simulink model "VSC_Grid"  (R2016b)
settings: Solver=VariableStepAuto  StartTime=0.0  StopTime=2  FixedStep=Ts  MaxStep=Ts  RelTol=1e-3  AbsTol=1e-3  EnableMultiTasking=on
undefined symbols (not defined in the file): alpha_PLL, alpha_PQ, DiscIntNeverNeededParam, fmax, fmin, fn, Ib, Kp_CC, Lf, Lf_pu, Rf, Sb, Ts, Vb, Vdcb, wn
libraries: powerlib x10, powerlib_meascontrol x10
Description:
  | Copyright 2008-2016 The MathWorks, Inc.
settings Model: FPTRunName=Active  ExtModeTrigMode=oneshot  ExtModeArmWhenConnect=off  ExtModeAutoUpdateStatusClock=off  Creator=MathWorks  LastModifiedBy=peiyuan
settings DataIOCC: SaveFormat=Array  SignalLoggingSaveFormat=ModelDataLogs  SaveOutput=off  SaveTime=off  SignalLoggingName=sigsOut
settings OptimizationCC: BlockReduction=off  BooleanDataType=off  ExpressionDepthLimit=2147483647  InitFltsAndDblsToZero=on  EfficientMapNaN2IntZero=off  LifeSpan=inf
settings DebuggingCC: SaveWithParameterizedLinksMsg=none  UnderspecifiedInitializationDetection=Classic  MergeDetectMultiDrivingBlocksExec=none  CheckExecutionContextPreStartOutputMsg=on  CheckExecutionContextRuntimeOutputMsg=on  SignalResolutionControl=TryResolveAllWithWarning  MultiTaskDSMMsg=warning  MultiTaskCondExecSysMsg=none  FcnCallInpInsideContextMsg=warning  AllowSymbolicDim=off  StateNameClashWarn=warning  SFUnexpectedBacktrackingDiag=warning  SFNoUnconditionalDefaultTransitionDiag=warning  SFExecutionAtInitializationDiag=none
settings HardwareCC: ProdBitPerPointer=32  ProdBitPerSizeT=32  ProdBitPerPtrDiffT=32  ProdLargestAtomicFloat=None  ProdIntDivRoundTo=Undefined  ProdEndianess=Unspecified  ProdWordSize=32  ProdHWDeviceType=32-bit Generic  TargetUnknown=on
settings ModelReferenceCC: PropagateSignalLabelsOutOfModel=off
settings GRTTargetCC: TargetFcnLib=ansi_tfl_tmw.mat  TargetLangStandard=C89/C90 (ANSI)  GeneratePreprocessorConditionals=Disable all  CombineOutputUpdateFcns=off  GRTInterface=on
settings ConfigComp: CovMetricSettings=dw  CovHtmlReporting=on  CovSaveCumulativeToWorkspaceVar=on  CovSaveSingleToWorkspaceVar=on  CovExternalEMLEnable=off  CovSFcnEnable=off

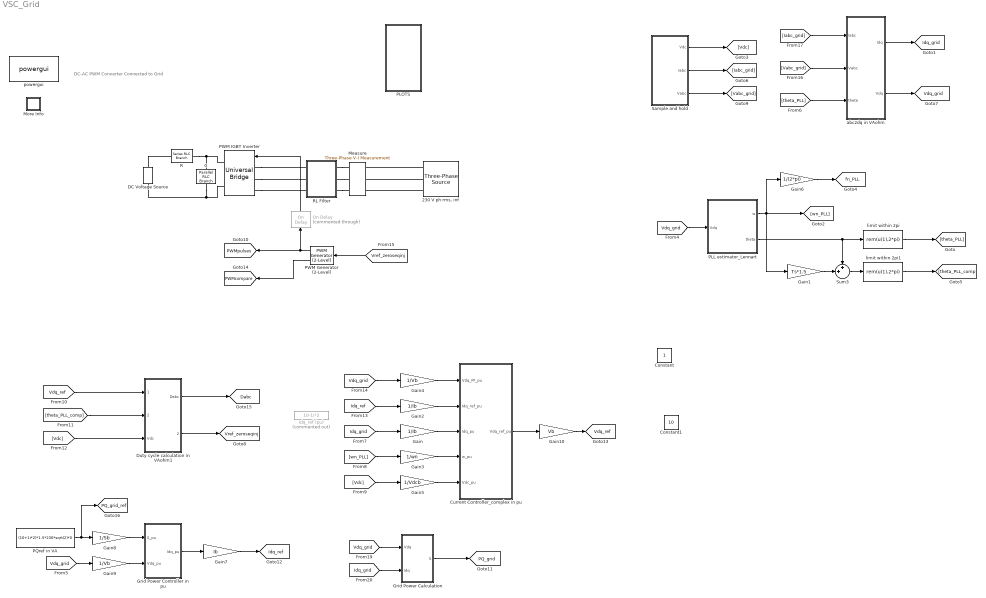
== system VSC_Grid ==
  note: DC-AC PWM Converter Connected to Grid
  "230 V ph rms, inf" : powerlib/Electrical Sources/Three-Phase Source  InternalConnection=Yg  VoltagePhases=off  Voltage=230*sqrt(3)  PhaseAngle=0  Voltage_phases=[25e3 25e3 25e3]/sqrt(3)  PhaseAngles_phases=[0 -120 +120]  Frequency=50  NonIdealSource=off  SpecifyImpedance=on  Resistance=0.8929  Inductance=16.58e-3  ShortCircuitLevel=40e6  BaseVoltage=600  XRratio=7  BusType=swing  Pref=0  Qref=0  Prefabc=[10e3, 10e3, 10e3]  Qrefabc=[0, 0, 0]  Qmin=-inf  Qmax=inf
  C : powerlib/Elements/Parallel RLC Branch  LConnTagsString=a  RConnTagsString=__new0  BranchType=C  Resistance=inf  Inductance=inf  SetiL0=off  InitialCurrent=0  Capacitance=5000e-06  Setx0=off  InitialVoltage=0  Measurements=Branch voltage
  Constant : Constant
  Constant1 : Constant  Value=10
  Current Controller_complex in pu : Subsystem
  DC Voltage Source : powerlib/Electrical Sources/DC Voltage Source  Amplitude=680  Measurements=None
  Duty cycle calculation in VAohm1 : Subsystem
  Gain : Gain  Gain=1/Ib
  Gain1 : Gain  Gain=Ts*1.5
  Gain10 : Gain  Gain=Vb
  Gain2 : Gain  Gain=1/Ib
  Gain3 : Gain  Gain=1/wn
  Gain4 : Gain  Gain=1/Vb
  Gain5 : Gain  Gain=1/Vdcb
  Gain6 : Gain  Gain=1/(2*pi)
  Gain7 : Gain  Gain=Ib
  Gain8 : Gain  Gain=1/Sb
  Gain9 : Gain  Gain=1/Vb
  Grid Power Calculation : Subsystem
  Grid Power Controller in pu : Subsystem
  Idq_ref (pu) : Constant  Commented=on  Value=10-1i*2
  Measure : powerlib/Measurements/Three-Phase V-I Measurement  VoltageMeasurement=phase-to-ground  SetLabelV=on  LabelV=Vabc_grid_analog  Vpu=off  VpuLL=off  CurrentMeasurement=yes  SetLabelI=on  LabelI=Iabc_grid_analog  Ipu=off  Pbase=Sb  Vbase=Vb*sqrt(3/2)  OutputType=Magnitude  PhasorSimulation=off  PSBequivalent=0
  More Info : Subsystem
      settings: OpenFcn=showdemo(bdroot(gcb))
      mask Display: disp('?')
  On Delay : powerlib_meascontrol/Logic/On Delay  Commented=through  DelayType=On delay  delay=0.01  ic=0  Ts=Ts
  PLL estimator_Lennart : Subsystem  mask(PLL estimator (discrete)){alpha_theta=alpha_PLL, fnmax=fmax, fnmin=fmin, f0=fn, Ts=Ts}
      mask prompts: alpha_theta "Bandwidth (natural freq, rad/s)"; fnmax "Max frequency (Hz)"; fnmin "Min frequency (Hz)"; f0 "Initial frequency (Hz)"; Ts "Sampling time (s)"
      mask help: The PLL is implemented according to Harnefors' paper, a second order system with critically damped case (damping ratio =1)
  PLOTS : Subsystem
  PQref in VA : Constant  Value=(10+1i*2)*1.5*230*sqrt(2)*0
  PWM IGBT Inverter : powerlib/Power Electronics/Universal Bridge  Arms=3  SnubberResistance=5000  SnubberCapacitance=inf  Device=IGBT / Diodes  Ron=1e-3  Lon=0  ForwardVoltages="[  0.0  0.0  ]"  ForwardVoltage=.8  GTOparameters=[ 1e-6 ,1e-6 ]  IGBTparameters=[ 1e-6 , 2e-6 ]  Measurements=All voltages and currents  Measurements_2=None  converterType=Rectifier
  PWM Generator (2-Level) : powerlib_meascontrol/Pulse & Signal Generators/PWM Generator (2-Level)  ModulatorType=Three-phase bridge (6 pulses)  ModulatorMode=Unsynchronized  Fc=5000  Pc=0  nF=27  MinMax="[ -1  1 ]"  SamplingTechnique=Symmetrical regular (single edge)  ModulatingSignals=off  m=0.8  Freq=60  Phase=0  Ts=0  ShowCarrierOutport=on
  R : powerlib/Elements/Series RLC Branch  LConnTagsString=__new0  RConnTagsString=__new0  BranchType=R  Resistance=1e-5  Inductance=1e-3  SetiL0=off  InitialCurrent=0  Capacitance=1e-6  Setx0=off  InitialVoltage=0  Measurements=None
  RL Filter : Subsystem
  Sample and hold : Subsystem
  Sum3 : Sum  Inputs=++|  SaturateOnIntegerOverflow=on  InputSameDT=on  OutDataTypeStr=Inherit: Same as first input
  abc2dq in VAohm : Subsystem
  limit within 2pi : Fcn  Expr=rem(u(1),2*pi)
  limit within 2pi1 : Fcn  Expr=rem(u(1),2*pi)
  powergui : powerlib/powergui  Priority=1  SimulationMode=Continuous  SolverType=Tustin/Backward Euler (TBE)  SampleTime=50e-6  frequency=60  SPID=off  DisableSnubberDevices=off  DisableRonSwitches=off  DisableVfSwitches=off  SwTol=0  DisplayEquations=off  Interpol=off  ExternalGateDelay=off  methode=off  Ts=10  FunctionMessages=off  echomessages=off  HookPort=off  EnableUseOfTLC=off  x0status=blocks  frequencyindice=50  Pbase=35e3  ErrMax=1e-4  Iterations=50  UnitsV=V  UnitsW=kW  buscounter=0  RestoreLinks=warning  ResistiveCurrentMeasurement=off  Frange=[0:2:500]  Ylog=off  Xlog=on  ShowGrid=off  save=off  variable=ZData  structure=0  ZoomFFT=off  StartTime=0.0  cycles=1  DisplayStyle=1  fundamental=60  FreqAxis=off  MaxFrequency=1000  frequencyindicesteady=1  RmsSteady=1  display=off
  tag scope: Dabc=global, Idq_grid=global, Idq_ref=global, PQ_grid=global, PQ_grid_ref=global, PWMcompare=global, PWMpulses=global, Vdq_grid=global, Vdq_ref=global, Vref_zeroseqinj=global, fn_PLL=global
  wires:
  On Delay/1 -> PWM IGBT Inverter/1
  PLL estimator_Lennart/2(theta) -> Sum3/1, limit within 2pi/1
  limit within 2pi/1 -> [theta_PLL]
  abc2dq in VAohm/1(Idq) -> [Idq_grid]
  [Vdq_grid] -> Gain4/1
  [Idq_grid] -> Gain/1
  [wn_PLL] -> Gain3/1
  [Vdc] -> Gain5/1
  Current Controller_complex in pu/1(Vdq_ref_pu) -> Gain10/1
  Gain1/1 -> Sum3/2
  Sum3/1 -> limit within 2pi1/1
  limit within 2pi1/1 -> [theta_PLL_comp]
  abc2dq in VAohm/2(Vdq) -> [Vdq_grid]
  [Vref_zeroseqinj] -> PWM Generator (2-Level)/1
  [Vdq_ref] -> Duty cycle calculation in VAohm1/1(Vdq_ref)
  [theta_PLL_comp] -> Duty cycle calculation in VAohm1/2(theta_comp)
  [Vdc] -> Duty cycle calculation in VAohm1/3(Vdc)
  Duty cycle calculation in VAohm1/1(Dabc) -> [Dabc]
  Duty cycle calculation in VAohm1/2(Vref_pu) -> [Vref_zeroseqinj]
  Gain3/1 -> Current Controller_complex in pu/4(w_pu)
  Gain/1 -> Current Controller_complex in pu/3(Idq_pu)
  Gain5/1 -> Current Controller_complex in pu/5(Vdc_pu)
  [theta_PLL] -> abc2dq in VAohm/3(theta)
  Gain4/1 -> Current Controller_complex in pu/1(Vdq_FF_pu)
  [Vdq_grid] -> PLL estimator_Lennart/1(Vdq)
  PLL estimator_Lennart/1(w) -> Gain6/1, Gain1/1, [wn_PLL]
  [Iabc_grid] -> abc2dq in VAohm/1(Iabc)
  [Vabc_grid] -> abc2dq in VAohm/2(Vabc)
  Gain6/1 -> [fn_PLL]
  Sample and hold/2(Iabc) -> [Iabc_grid]
  Sample and hold/3(Vabc) -> [Vabc_grid]
  PQref in VA/1 -> [PQ_grid_ref], Gain8/1
  [Vdq_grid] -> Gain9/1
  Gain8/1 -> Grid Power Controller in pu/1(S_pu)
  Gain9/1 -> Grid Power Controller in pu/2(Vdq_pu)
  Grid Power Controller in pu/1(Idq_pu) -> Gain7/1
  [Vdq_grid] -> Grid Power Calculation/1(Vdq)
  Grid Power Calculation/1(S) -> [PQ_grid]
  [Idq_grid] -> Grid Power Calculation/2(Idq)
  Gain7/1 -> [Idq_ref]
  Gain10/1 -> [Vdq_ref]
  Gain2/1 -> Current Controller_complex in pu/2(Idq_ref_pu)
  [Idq_ref] -> Gain2/1
  PWM Generator (2-Level)/1 -> [PWMpulses], On Delay/1
  PWM Generator (2-Level)/2 -> [PWMcompare]
  Sample and hold/1(Vdc) -> [Vdc]
  connections:
  PWM IGBT Inverter/RConn2 -- DC Voltage Source/LConn1 -- C/RConn1
  R/RConn1 -- C/LConn1 -- PWM IGBT Inverter/RConn1
  RL Filter/RConn1 -- Measure/LConn1
  Measure/LConn2 -- RL Filter/RConn2
  RL Filter/RConn3 -- Measure/LConn3
  PWM IGBT Inverter/LConn2 -- RL Filter/LConn2
  PWM IGBT Inverter/LConn3 -- RL Filter/LConn3
  PWM IGBT Inverter/LConn1 -- RL Filter/LConn1
  "230 V ph rms, inf"/RConn2 -- Measure/RConn2
  "230 V ph rms, inf"/RConn1 -- Measure/RConn1
  R/LConn1 -- DC Voltage Source/RConn1
  "230 V ph rms, inf"/RConn3 -- Measure/RConn3

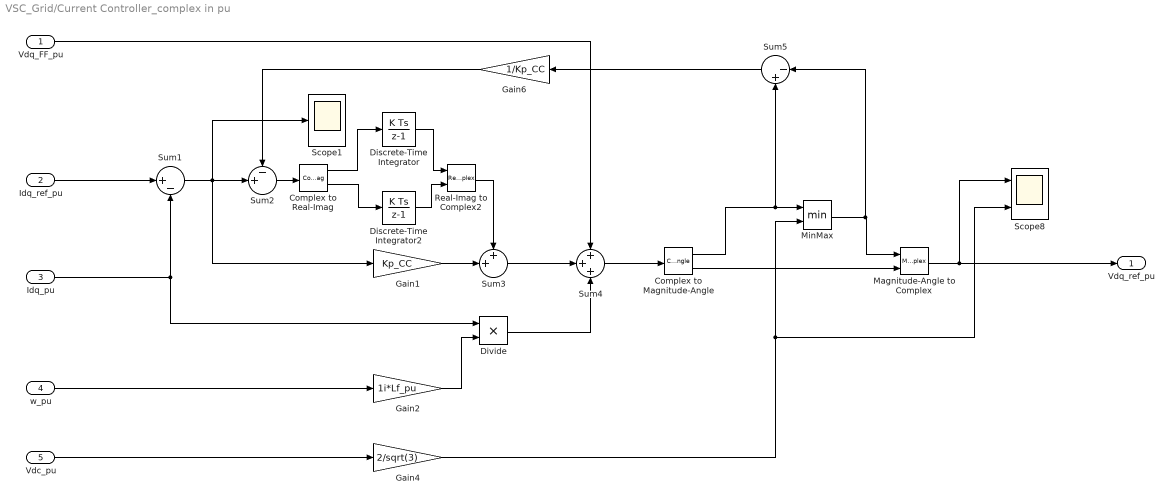
== system VSC_Grid/Current Controller_complex in pu ==
  Vdq_FF_pu : Inport
  Idq_ref_pu : Inport  Port=2
  Idq_pu : Inport  Port=3
  w_pu : Inport  Port=4
  Vdc_pu : Inport  Port=5
  Complex to Magnitude-Angle : ComplexToMagnitudeAngle
  Complex to Real-Imag : ComplexToRealImag
  Discrete-Time Integrator : DiscreteIntegrator  gainval=Ki_CC  InitialConditionSetting=State (most efficient)  SampleTime=Ts  ICPrevOutput=DiscIntNeverNeededParam  ICPrevScaledInput=DiscIntNeverNeededParam
  Discrete-Time Integrator2 : DiscreteIntegrator  gainval=Ki_CC  InitialConditionSetting=State (most efficient)  SampleTime=Ts  ICPrevOutput=DiscIntNeverNeededParam  ICPrevScaledInput=DiscIntNeverNeededParam
  Divide : Product  Inputs=**
  Gain1 : Gain  Gain=Kp_CC
  Gain2 : Gain  Gain=1i*Lf_pu
  Gain4 : Gain  Gain=2/sqrt(3)
  Gain6 : Gain  Gain=1/Kp_CC
  Magnitude-Angle to Complex : MagnitudeAngleToComplex
  MinMax : MinMax  Inputs=2
  Real-Imag to Complex2 : RealImagToComplex
  Scope1 : Scope
  Scope8 : Scope  NumInputPorts=2
  Sum1 : Sum  Inputs=|+-  SaturateOnIntegerOverflow=on  InputSameDT=on  OutDataTypeStr=Inherit: Same as first input
  Sum2 : Sum  Inputs=-+|  SaturateOnIntegerOverflow=on  InputSameDT=on  OutDataTypeStr=Inherit: Same as first input
  Sum3 : Sum  Inputs=++|  SaturateOnIntegerOverflow=on  InputSameDT=on  OutDataTypeStr=Inherit: Same as first input
  Sum4 : Sum  Inputs=+++  SaturateOnIntegerOverflow=on  InputSameDT=on  OutDataTypeStr=Inherit: Same as first input
  Sum5 : Sum  Inputs=|-+  SaturateOnIntegerOverflow=on  InputSameDT=on  OutDataTypeStr=Inherit: Same as first input
  Vdq_ref_pu : Outport
  wires:
  Discrete-Time Integrator2/1 -> Real-Imag to Complex2/2
  Discrete-Time Integrator/1 -> Real-Imag to Complex2/1
  Complex to Real-Imag/2 -> Discrete-Time Integrator2/1
  Real-Imag to Complex2/1 -> Sum3/1
  Complex to Magnitude-Angle/2 -> Magnitude-Angle to Complex/2
  Sum5/1 -> Gain6/1
  Gain4/1 -> Scope8/2, MinMax/2
  Complex to Real-Imag/1 -> Discrete-Time Integrator/1
  Idq_pu/1 -> Divide/1, Sum1/2
  Divide/1 -> Sum4/3
  Idq_ref_pu/1 -> Sum1/1
  Sum4/1 -> Complex to Magnitude-Angle/1
  Sum1/1 -> Scope1/1, Gain1/1, Sum2/2
  Gain2/1 -> Divide/2
  Complex to Magnitude-Angle/1 -> Sum5/2, MinMax/1
  Gain1/1 -> Sum3/2
  Sum3/1 -> Sum4/2
  w_pu/1 -> Gain2/1
  Vdq_FF_pu/1 -> Sum4/1
  Magnitude-Angle to Complex/1 -> Vdq_ref_pu/1, Scope8/1
  Sum2/1 -> Complex to Real-Imag/1
  MinMax/1 -> Sum5/1, Magnitude-Angle to Complex/1
  Gain6/1 -> Sum2/1
  Vdc_pu/1 -> Gain4/1

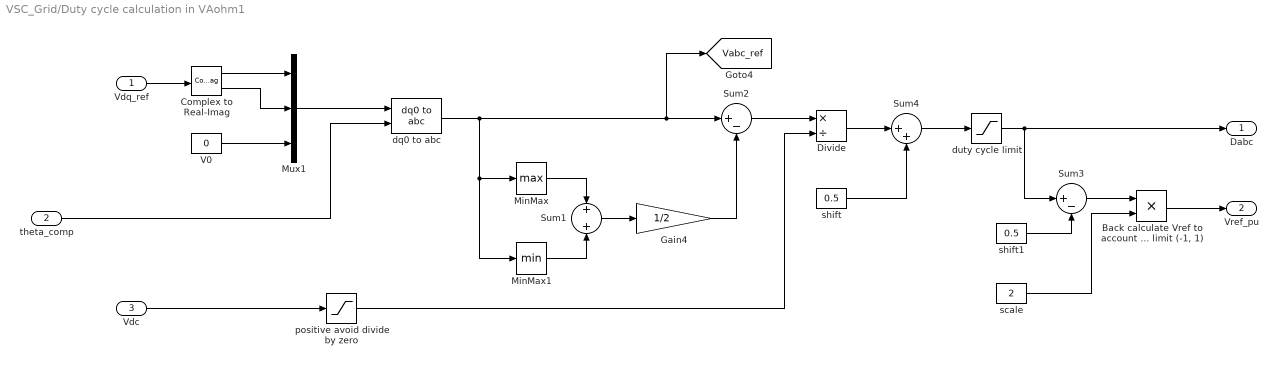
== system VSC_Grid/Duty cycle calculation in VAohm1 ==
  Vdq_ref : Inport
  theta_comp : Inport  Port=2
  Vdc : Inport  Port=3
  "Back calculate Vref to account for duty cycle limit (-1, 1)" : Product  Inputs=**
  Complex to Real-Imag : ComplexToRealImag
  Divide : Product  Inputs=*/
  Gain4 : Gain  Gain=1/2
  MinMax : MinMax  Function=max
  MinMax1 : MinMax
  Mux1 : Mux  Inputs=3
  Sum1 : Sum  SaturateOnIntegerOverflow=on  InputSameDT=on  OutDataTypeStr=Inherit: Same as first input
  Sum2 : Sum  Inputs=|+-  SaturateOnIntegerOverflow=on  InputSameDT=on  OutDataTypeStr=Inherit: Same as first input
  Sum3 : Sum  Inputs=|+-  SaturateOnIntegerOverflow=on  InputSameDT=on  OutDataTypeStr=Inherit: Same as first input
  Sum4 : Sum  Inputs=|++  SaturateOnIntegerOverflow=on  InputSameDT=on  OutDataTypeStr=Inherit: Same as first input
  V0 : Constant  Value=0
  dq0 to abc : powerlib_meascontrol/Transformations/dq0 to abc  Alignment=90 degrees behind phase A axis
  duty cycle limit : Saturate  UpperLimit=0.999  LowerLimit=0.001
  positive avoid divide by zero : Saturate  UpperLimit=inf  LowerLimit=1e-6
  scale : Constant  Value=2
  shift : Constant  Value=0.5
  shift1 : Constant  Value=0.5
  Dabc : Outport
  Vref_pu : Outport  Port=2
  tag scope: Vabc_ref=global
  wires:
  Sum2/1 -> Divide/1
  Gain4/1 -> Sum2/2
  dq0 to abc/1 -> MinMax/1, MinMax1/1, [Vabc_ref], Sum2/1
  MinMax1/1 -> Sum1/2
  shift/1 -> Sum4/2
  Vdq_ref/1 -> Complex to Real-Imag/1
  Complex to Real-Imag/2 -> Mux1/2
  Mux1/1 -> dq0 to abc/1
  Sum1/1 -> Gain4/1
  Divide/1 -> Sum4/1
  Vdc/1 -> positive avoid divide by zero/1
  theta_comp/1 -> dq0 to abc/2
  V0/1 -> Mux1/3
  MinMax/1 -> Sum1/1
  Complex to Real-Imag/1 -> Mux1/1
  Sum4/1 -> duty cycle limit/1
  duty cycle limit/1 -> Sum3/1, Dabc/1
  shift1/1 -> Sum3/2
  Sum3/1 -> "Back calculate Vref to account for duty cycle limit (-1, 1)"/1
  "Back calculate Vref to account for duty cycle limit (-1, 1)"/1 -> Vref_pu/1
  positive avoid divide by zero/1 -> Divide/2
  scale/1 -> "Back calculate Vref to account for duty cycle limit (-1, 1)"/2

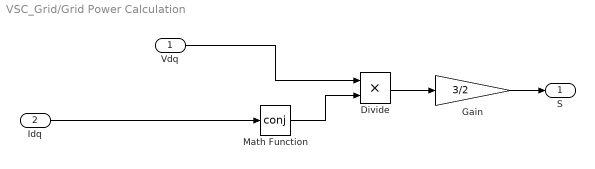
== system VSC_Grid/Grid Power Calculation ==
  Vdq : Inport
  Idq : Inport  Port=2
  Divide : Product  Inputs=**
  Gain : Gain  Gain=3/2
  Math Function : Math  Operator=conj  SaturateOnIntegerOverflow=on
  S : Outport
  wires:
  Idq/1 -> Math Function/1
  Math Function/1 -> Divide/2
  Divide/1 -> Gain/1
  Vdq/1 -> Divide/1
  Gain/1 -> S/1

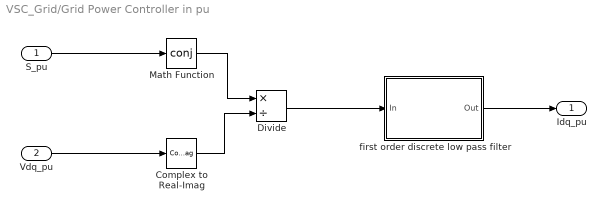
== system VSC_Grid/Grid Power Controller in pu ==
  S_pu : Inport
  Vdq_pu : Inport  Port=2
  Complex to Real-Imag : ComplexToRealImag  Output=Real
  Divide : Product  Inputs=*/
  Math Function : Math  Operator=conj  SaturateOnIntegerOverflow=on
  first order discrete low pass filter : Subsystem  mask(First-order low pass filter (Discrete)){alpha_wfilter=alpha_PQ, Ts=Ts, Init=(10-1i*2)/Ib*0}
      mask prompts: alpha_wfilter "Bandwidth (rad/s)"; Ts "Sampling time (>0, s)"; Init "Initial condition"
      mask help: Forward Euler method
  Idq_pu : Outport
  wires:
  Vdq_pu/1 -> Complex to Real-Imag/1
  Complex to Real-Imag/1 -> Divide/2
  S_pu/1 -> Math Function/1
  Math Function/1 -> Divide/1
  Divide/1 -> first order discrete low pass filter/1(In)
  first order discrete low pass filter/1(Out) -> Idq_pu/1

== system VSC_Grid/More Info ==

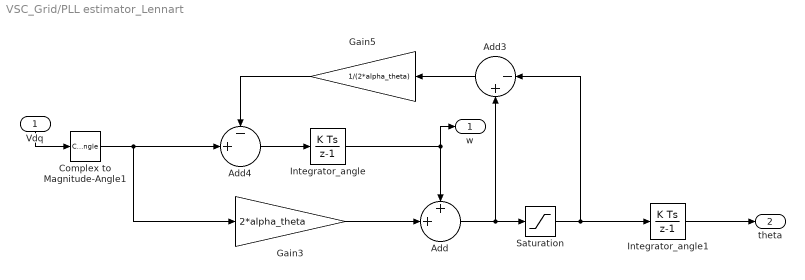
== system VSC_Grid/PLL estimator_Lennart ==
  Vdq : Inport
  Add : Sum  Inputs=++|
  Add3 : Sum  Inputs=|-+
  Add4 : Sum  Inputs=-+|
  Complex to Magnitude-Angle1 : ComplexToMagnitudeAngle  Output=Angle
  Gain3 : Gain  Gain=2*alpha_theta
  Gain5 : Gain  Gain=1/(2*alpha_theta)
  Integrator_angle : DiscreteIntegrator  gainval=alpha_theta^2  InitialCondition=2*pi*f0  InitialConditionSetting=State (most efficient)  SampleTime=Ts  ICPrevOutput=DiscIntNeverNeededParam  ICPrevScaledInput=DiscIntNeverNeededParam
  Integrator_angle1 : DiscreteIntegrator  gainval=1  InitialConditionSetting=State (most efficient)  SampleTime=Ts  ICPrevOutput=DiscIntNeverNeededParam  ICPrevScaledInput=DiscIntNeverNeededParam
  Saturation : Saturate  UpperLimit=2*pi*fnmax  LowerLimit=2*pi*fnmin
  w : Outport
  theta : Outport  Port=2
  wires:
  Integrator_angle1/1 -> theta/1
  Gain5/1 -> Add4/1
  Gain3/1 -> Add/2
  Add/1 -> Add3/2, Saturation/1
  Vdq/1 -> Complex to Magnitude-Angle1/1
  Integrator_angle/1 -> w/1, Add/1
  Add3/1 -> Gain5/1
  Add4/1 -> Integrator_angle/1
  Saturation/1 -> Integrator_angle1/1, Add3/1
  Complex to Magnitude-Angle1/1 -> Gain3/1, Add4/2

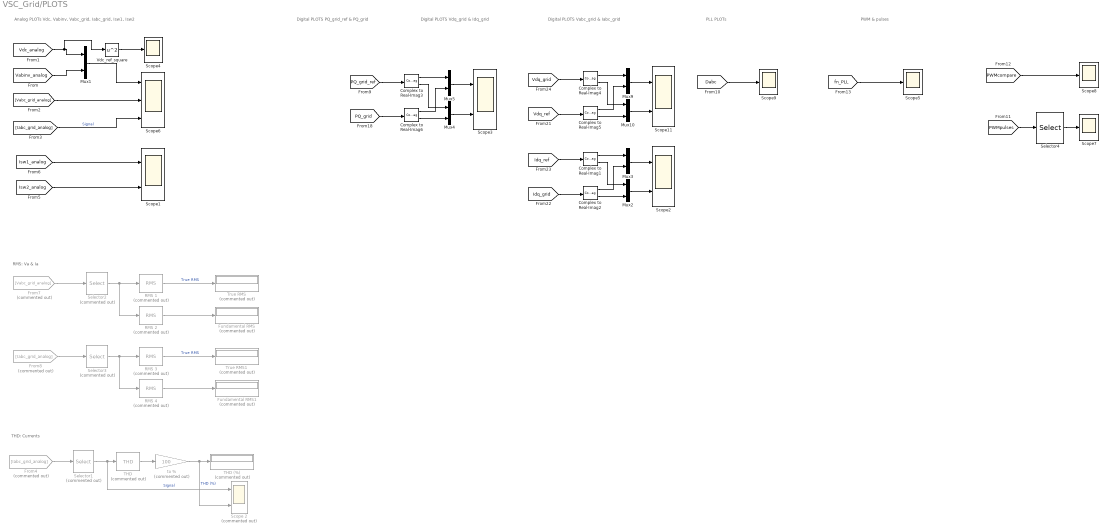
== system VSC_Grid/PLOTS ==
  note: Digital PLOTS
      | Vdq_grid & Idq_grid
  note: Analog PLOTs
      | Vdc, Vabinv, Vabc_grid, Iabc_grid, Isw1, Isw2
  note: THD: Currents
  note: RMS: Va & Ia
  note: PLL PLOTs
  note: Digital PLOTS
      | Vabc_grid & Iabc_grid
  note: PWM & pulses
  note: Digital PLOTS
      | PQ_grid_ref & PQ_grid
  Complex to Real-Imag{1..6} (6 alike) : ComplexToRealImag
  From4 : From  Commented=on  GotoTag=Iabc_grid_analog  TagVisibility=global
  From7 : From  Commented=on  GotoTag=Vabc_grid_analog  TagVisibility=global
  From8 : From  Commented=on  GotoTag=Iabc_grid_analog  TagVisibility=global
  Fundamental RMS : Display  Commented=on
      settings: Format=bank
  Fundamental RMS1 : Display  Commented=on
      settings: Format=bank
  Mux{1..5,9..10} (7 alike) : Mux  Inputs=2
  RMS 1 : powerlib_meascontrol/Measurements/RMS  Commented=on  TrueRMS=on  Freq=fn  RMSInit=Vb  Ts=0
  RMS 2 : powerlib_meascontrol/Measurements/RMS  Commented=on  TrueRMS=off  Freq=fn  RMSInit=Vb  Ts=0
  RMS 3 : powerlib_meascontrol/Measurements/RMS  Commented=on  TrueRMS=on  Freq=fn  RMSInit=Ib  Ts=0
  RMS 4 : powerlib_meascontrol/Measurements/RMS  Commented=on  TrueRMS=off  Freq=fn  RMSInit=Ib  Ts=0
  Scope 2 : Scope  Commented=on  NumInputPorts=2
  Scope{1..3,11} (4 alike) : Scope  NumInputPorts=2
  Scope{4..5,7..9} (5 alike) : Scope
  Scope6 : Scope  NumInputPorts=3
  Selector1 : Selector  Commented=on  InputPortWidth=3  IndexOptions=Index vector (dialog)  Indices=[1]  OutputSizes=1
  Selector2 : Selector  Commented=on  InputPortWidth=3  IndexOptions=Index vector (dialog)  Indices=[1]  OutputSizes=1
  Selector3 : Selector  Commented=on  InputPortWidth=3  IndexOptions=Index vector (dialog)  Indices=[1]  OutputSizes=1
  Selector4 : Selector  InputPortWidth=6  IndexOptions=Index vector (dialog)  Indices=[1]  OutputSizes=1
  THD : powerlib_meascontrol/Measurements/THD  Commented=on  Freq=50  Ts=0
  THD (%) : Display  Commented=on
      settings: Format=bank
  True RMS : Display  Commented=on
      settings: Format=bank
  True RMS1 : Display  Commented=on
      settings: Format=bank
  Vdc_ref_square : Math  Operator=square  SaturateOnIntegerOverflow=on
  to % : Gain  Commented=on  Gain=100  SampleTime=Ts
  wires:
  [Iabc_grid_analog] -> Scope6/3  "Signal"
  to %/1 -> THD (%)/1, Scope 2/2  "THD (%)"
  THD/1 -> to %/1
  [Vdc_analog] -> Vdc_ref_square/1, Mux1/1
  [Vabinv_analog] -> Mux1/2
  Mux1/1 -> Scope6/1
  [Vabc_grid_analog] -> Scope6/2
  [Isw1_analog] -> Scope1/1
  [Isw2_analog] -> Scope1/2
  From4/1 -> Selector1/1
  Selector1/1 -> THD/1, Scope 2/1  "Signal"
  RMS 1/1 -> True RMS/1  "True RMS"
  From7/1 -> Selector2/1
  Selector2/1 -> RMS 2/1, RMS 1/1
  RMS 2/1 -> Fundamental RMS/1
  RMS 3/1 -> True RMS1/1  "True RMS"
  Selector3/1 -> RMS 4/1, RMS 3/1
  RMS 4/1 -> Fundamental RMS1/1
  From8/1 -> Selector3/1
  Vdc_ref_square/1 -> Scope4/1
  [fn_PLL] -> Scope5/1
  [Dabc] -> Scope9/1
  Selector4/1 -> Scope7/1
  [PWMpulses] -> Selector4/1
  [PWMcompare] -> Scope8/1
  Complex to Real-Imag4/1 -> Mux9/1
  Complex to Real-Imag5/1 -> Mux9/2
  Complex to Real-Imag4/2 -> Mux10/1
  Complex to Real-Imag5/2 -> Mux10/2
  Mux9/1 -> Scope11/1
  Mux10/1 -> Scope11/2
  Complex to Real-Imag1/1 -> Mux3/1
  Complex to Real-Imag2/1 -> Mux3/2
  Complex to Real-Imag1/2 -> Mux2/1
  Complex to Real-Imag2/2 -> Mux2/2
  Mux3/1 -> Scope2/1
  Mux2/1 -> Scope2/2
  [Idq_ref] -> Complex to Real-Imag1/1
  [Idq_grid] -> Complex to Real-Imag2/1
  [Vdq_grid] -> Complex to Real-Imag4/1
  [Vdq_ref] -> Complex to Real-Imag5/1
  Complex to Real-Imag3/1 -> Mux5/1
  Complex to Real-Imag6/1 -> Mux5/2
  Complex to Real-Imag3/2 -> Mux4/1
  Complex to Real-Imag6/2 -> Mux4/2
  Mux5/1 -> Scope3/1
  Mux4/1 -> Scope3/2
  [PQ_grid_ref] -> Complex to Real-Imag3/1
  [PQ_grid] -> Complex to Real-Imag6/1

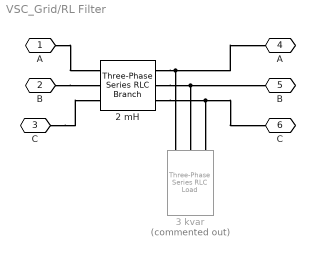
== system VSC_Grid/RL Filter ==
  "2 mH " : powerlib/Elements/Three-Phase Series RLC Branch  LConnTagsString=A|B|C  RConnTagsString=A|B|C  BranchType=RL  Resistance=Rf  Inductance=Lf  Capacitance=inf  Measurements=None
  3 kvar : powerlib/Elements/Three-Phase Series RLC Load  Commented=on  LConnTagsString=A|B|C  Configuration=Y (grounded)  NominalVoltage=380  Vabc=[1e3 1e3 1e3]  Vabcp=[1e3 1e3 1e3]  NominalFrequency=50  UnbalancedPower=off  ActivePower=0  InductivePower=0  CapacitivePower=3e3  Pabc=[10e3 9e3 11e3]  QLabc=[100 90 110]  QCabc=[100 90 110]  Pabcp=[10e3 9e3 11e3]  QLabcp=[100 90 110]  QCabcp=[100 90 110]  Measurements=None  LoadType=constant Z
  A : PMIOPort  Port=1  Side=Left
  B : PMIOPort  Port=2  Side=Left
  C : PMIOPort  Port=3  Side=Left
  "A " : PMIOPort  Port=4  Side=Right
  "B " : PMIOPort  Port=5  Side=Right
  "C " : PMIOPort  Port=6  Side=Right
  connections:
  B/RConn1 -- "2 mH "/LConn2
  A/RConn1 -- "2 mH "/LConn1
  C/RConn1 -- "2 mH "/LConn3
  "2 mH "/RConn1 -- "A "/RConn1 -- 3 kvar/LConn1
  "2 mH "/RConn2 -- "B "/RConn1 -- 3 kvar/LConn2
  "2 mH "/RConn3 -- "C "/RConn1 -- 3 kvar/LConn3

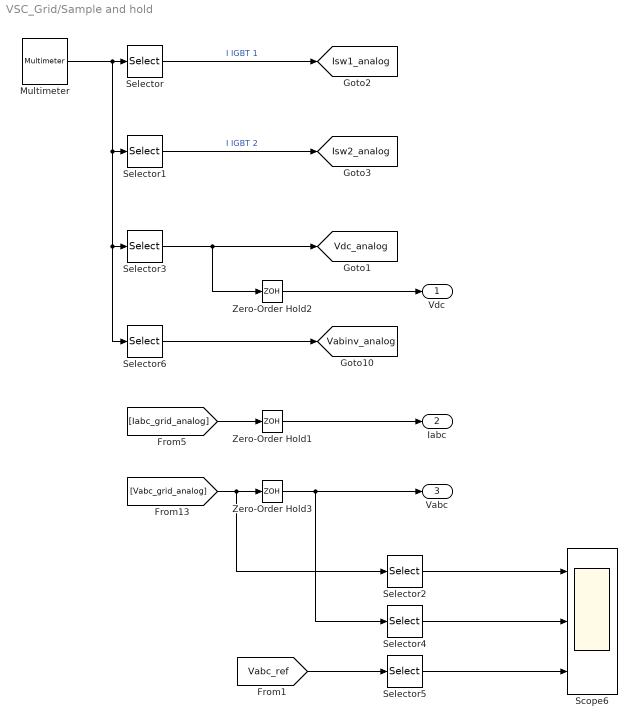
== system VSC_Grid/Sample and hold ==
  Multimeter : powerlib/Measurements/Multimeter  Tag=PoWeRsYsTeMmEaSuReMeNt  PhasorSimulation=off  OutputType=Magnitude  sel=[12 13 1 8]  L=17  Gain=[1 1 1 1]  yselected="{'Isw1: PWM  IGBT Inverter','Isw2: PWM  IGBT Inverter','Ub: C','Uab: PWM  IGBT Inverter'};"  PSBOutputType=1  PSBequivalent=0  AxesSetting=[0,0.1,-100,100]  Display=0  SavedBlockNames=-11
      settings: AttributesFormatString=\n
  Scope6 : Scope  NumInputPorts=3
  Selector : Selector  InputPortWidth=4  IndexOptions=Index vector (dialog)  Indices=[1]  OutputSizes=1
  Selector1 : Selector  InputPortWidth=4  IndexOptions=Index vector (dialog)  Indices=[2]  OutputSizes=1
  Selector2 : Selector  InputPortWidth=3  IndexOptions=Index vector (dialog)  Indices=[1]  OutputSizes=1
  Selector3 : Selector  InputPortWidth=4  IndexOptions=Index vector (dialog)  Indices=[3]  OutputSizes=1
  Selector4 : Selector  InputPortWidth=3  IndexOptions=Index vector (dialog)  Indices=[1]  OutputSizes=1
  Selector5 : Selector  InputPortWidth=3  IndexOptions=Index vector (dialog)  Indices=[1]  OutputSizes=1
  Selector6 : Selector  InputPortWidth=4  IndexOptions=Index vector (dialog)  Indices=[4]  OutputSizes=1
  Zero-Order Hold1 : ZeroOrderHold  SampleTime=Ts
  Zero-Order Hold2 : ZeroOrderHold  SampleTime=Ts
  Zero-Order Hold3 : ZeroOrderHold  SampleTime=Ts
  Vdc : Outport
  Iabc : Outport  Port=2
  Vabc : Outport  Port=3
  tag scope: Isw1_analog=global, Isw2_analog=global, Vabinv_analog=global, Vdc_analog=global
  wires:
  [Iabc_grid_analog] -> Zero-Order Hold1/1
  Zero-Order Hold3/1 -> Selector4/1, Vabc/1
  Zero-Order Hold1/1 -> Iabc/1
  [Vabc_grid_analog] -> Selector2/1, Zero-Order Hold3/1
  Selector2/1 -> Scope6/1
  Selector4/1 -> Scope6/2
  [Vabc_ref] -> Selector5/1
  Selector5/1 -> Scope6/3
  Selector/1 -> [Isw1_analog]  "I IGBT 1"
  Multimeter/1 -> Selector/1, Selector6/1, Selector3/1, Selector1/1
  Selector3/1 -> [Vdc_analog], Zero-Order Hold2/1
  Selector6/1 -> [Vabinv_analog]
  Selector1/1 -> [Isw2_analog]  "I IGBT 2"
  Zero-Order Hold2/1 -> Vdc/1

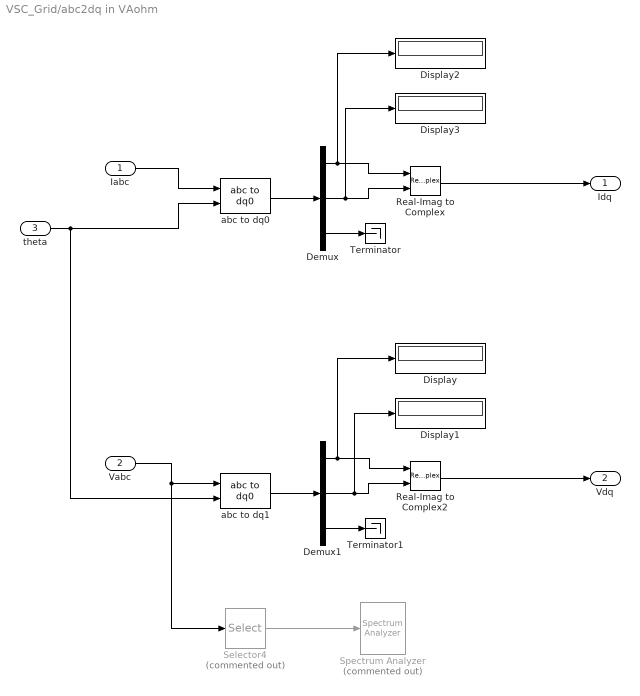
== system VSC_Grid/abc2dq in VAohm ==
  Iabc : Inport
  Vabc : Inport  Port=2
  theta : Inport  Port=3
  Demux : Demux  Outputs=3
  Demux1 : Demux  Outputs=3
  Display{,1..3} (4 alike) : Display
  Real-Imag to Complex : RealImagToComplex
  Real-Imag to Complex2 : RealImagToComplex
  Selector4 : Selector  Commented=on  InputPortWidth=3  IndexOptions=Index vector (dialog)  Indices=[1]  OutputSizes=1
  Spectrum Analyzer : SpectrumAnalyzer  Commented=on
  Terminator : Terminator
  Terminator1 : Terminator
  abc to dq0 : powerlib_meascontrol/Transformations/abc to dq0  Alignment=90 degrees behind phase A axis
  abc to dq1 : powerlib_meascontrol/Transformations/abc to dq0  Alignment=90 degrees behind phase A axis
  Idq : Outport
  Vdq : Outport  Port=2
  wires:
  Demux1/1 -> Display/1, Real-Imag to Complex2/1
  theta/1 -> abc to dq1/2, abc to dq0/2
  Vabc/1 -> abc to dq1/1, Selector4/1
  abc to dq1/1 -> Demux1/1
  Demux1/3 -> Terminator1/1
  Demux1/2 -> Display1/1, Real-Imag to Complex2/2
  Real-Imag to Complex2/1 -> Vdq/1
  Selector4/1 -> Spectrum Analyzer/1
  Iabc/1 -> abc to dq0/1
  abc to dq0/1 -> Demux/1
  Demux/1 -> Display2/1, Real-Imag to Complex/1
  Real-Imag to Complex/1 -> Idq/1
  Demux/2 -> Display3/1, Real-Imag to Complex/2
  Demux/3 -> Terminator/1

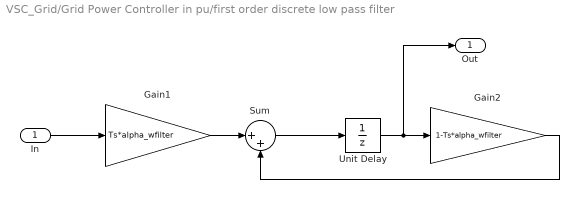
== system VSC_Grid/Grid Power Controller in pu/first order discrete low pass filter ==
  In : Inport
  Gain1 : Gain  Gain=Ts*alpha_wfilter
  Gain2 : Gain  Gain=1-Ts*alpha_wfilter
  Sum : Sum  Inputs=|++
  Unit Delay : UnitDelay  InitialCondition=Init  SampleTime=Ts
  Out : Outport
  wires:
  Gain2/1 -> Sum/2
  In/1 -> Gain1/1
  Sum/1 -> Unit Delay/1
  Gain1/1 -> Sum/1
  Unit Delay/1 -> Out/1, Gain2/1
